simulink model "temp_motor_model"  (R2022b)
settings: Solver=ode45  StartTime=0.0  StopTime=1.0  RelTol=1e-3
values from neighbouring files (symbols this model uses):
  k_sim = k_all(i)    [full_old.m]    (also in m_code_lab_1.m)
  Tm_sim = Tm_all(i)    [full_old.m]    (also in m_code_lab_1.m)
  U_sim = U_pr    [full_old.m]    (also in m_code_lab_1.m)
settings Model: Creator=Eternal_Core  LastModifiedBy=Eternal_Core

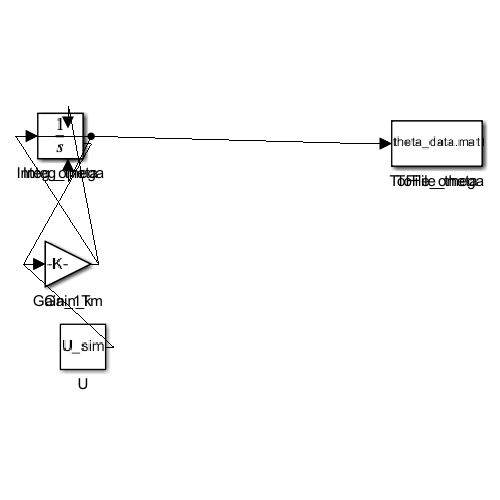
[thumbnail: Simulink's stored preview of the top-level diagram]
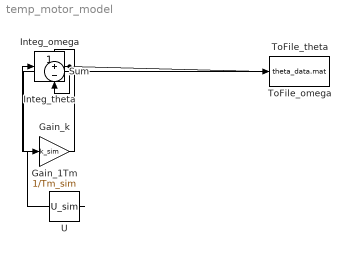
== system temp_motor_model ==
  Gain_1Tm : Gain  Gain=1/Tm_sim
  Gain_k : Gain  Gain=k_sim
  Integ_omega : Integrator
  Integ_theta : Integrator
  Sum : Sum  Inputs=+-
  ToFile_omega : ToFile  Filename=omega_data.mat  SaveFormat=Timeseries
  ToFile_theta : ToFile  Filename=theta_data.mat  SaveFormat=Timeseries
  U : Constant  Value=U_sim
  wires:
  U/1 -> Gain_k/1
  Gain_k/1 -> Sum/1
  Integ_omega/1 -> Sum/2, Integ_theta/1, ToFile_omega/1
  Sum/1 -> Gain_1Tm/1
  Gain_1Tm/1 -> Integ_omega/1
  Integ_theta/1 -> ToFile_theta/1
